simulink model "DGL2_02"  (R2018a)
settings: Solver=VariableStepAuto  StartTime=0.0  StopTime=10.0  RelTol=1e-3
values from neighbouring files (symbols this model uses):
  A1 = [0   -g/L ... (first row only)    [test_simulink.m]    (also in ueb_simulink_Pendel.m)
  B1 = [0 0]'    [test_simulink.m]    (also in ueb_simulink_Pendel.m)
  C1 = [1 0 ... (first row only)    [test_simulink.m]    (also in ueb_simulink_Pendel.m)
  D1 = [0 0]'    [test_simulink.m]    (also in ueb_simulink_Pendel.m)
  u_in = 1    [test_simulink.m]
  x1_0 = [Omega_0 Phi_0]'    [test_simulink.m]    (also in ueb_simulink_Pendel.m)
settings Model: Creator=Horst  LastModifiedBy=Horst

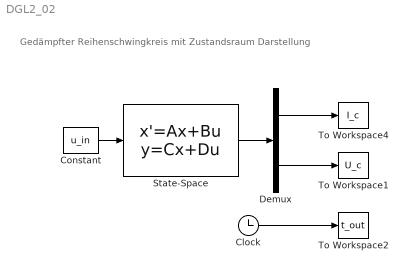
== system DGL2_02 ==
  note: Gedämpfter Reihenschwingkreis mit Zustandsraum Darstellung
  Clock : Clock
  Constant : Constant  Value=u_in
  Demux : Demux  Outputs=2
  State-Space : StateSpace  A=A1  B=B1  C=C1  D=D1  InitialCondition=x1_0
  To Workspace1 : ToWorkspace  VariableName=U_c  SampleTime=-1
  To Workspace2 : ToWorkspace  VariableName=t_out  SampleTime=-1
  To Workspace4 : ToWorkspace  VariableName=I_c  SampleTime=-1
  wires:
  Clock/1 -> To Workspace2/1
  Constant/1 -> State-Space/1
  Demux/1 -> To Workspace4/1
  Demux/2 -> To Workspace1/1
  State-Space/1 -> Demux/1
